simulink model "lookup_nD_TestGen25"  (R2017b)
settings: Solver=FixedStepDiscrete  StartTime=0.0  StopTime=10.0  RelTol=1e-3
settings Model: Creator=ktrinh  LastModifiedBy=ktrinh
settings DebuggingCC: ParameterOverflowMsg=none

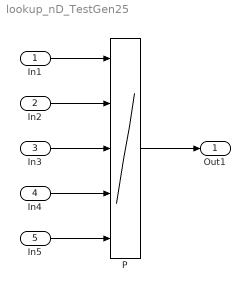
== system lookup_nD_TestGen25 ==
  In1 : Inport  OutMin=0  OutMax=127  OutDataTypeStr=uint16  PortDimensions=1
  In2 : Inport  Port=2  OutMin=0  OutMax=127  OutDataTypeStr=uint16
  In3 : Inport  Port=3  OutMin=0  OutMax=127  OutDataTypeStr=uint16
  In4 : Inport  Port=4  OutMin=0  OutMax=127  OutDataTypeStr=uint16
  In5 : Inport  Port=5  OutMin=0  OutMax=127  OutDataTypeStr=uint16
  P : Lookup_n-D  NumberOfTableDimensions=5  BreakpointsForDimension1=[49.7883202308942;52.545593266823]  BreakpointsForDimension2=[13.1724200537824;16.6042894722249;26.6818040792021;34.9361207449651;102.051615338463]  BreakpointsForDimension3=[28.9960950722709;62.130377382721;90.9645774641254]  BreakpointsForDimension4=[27.9367975156089;93.3623465556457]  BreakpointsForDimension5=[17.2229818359364;62.5382240354051;95.0077930063622]  BreakpointsForDimension1DataTypeStr=uint8  BreakpointsForDimension2DataTypeStr=uint8  BreakpointsForDimension3DataTypeStr=uint8  BreakpointsForDimension4DataTypeStr=uint8  BreakpointsForDimension5DataTypeStr=uint8  Table=reshape(repmat([4 5 6 7 8;16 19 20 21 22;10 18 23 24 25],6,2),[2,5,3,2,3])  TableDataTypeStr=Inherit: Inherit from 'Table data'  InterpMethod=Flat  ExtrapMethod=Clip  InternalRulePriority=Speed  OutDataTypeStr=uint8  RndMeth=Round  SaturateOnIntegerOverflow=on  InputSameDT=on
  Out1 : Outport
  wires:
  In1/1 -> P/1
  In2/1 -> P/2
  In3/1 -> P/3
  In4/1 -> P/4
  In5/1 -> P/5
  P/1 -> Out1/1
